simulink model "train_fuzzy4"  (R2017b)
settings: Solver=FixedStepAuto  StartTime=0.0  StopTime=1000  FixedStep=0.01  RelTol=1e-3
libraries: fuzblock x1
settings Model: Creator=QuocViet  LastModifiedBy=QuocViet
settings DebuggingCC: UnconnectedInputMsg=none  UnconnectedOutputMsg=none  UnconnectedLineMsg=none  SFMachineParentedDataDiag=error
settings SFSimCC: SimUseLocalCustomCode=on
settings RTWCC: RTWUseLocalCustomCode=on

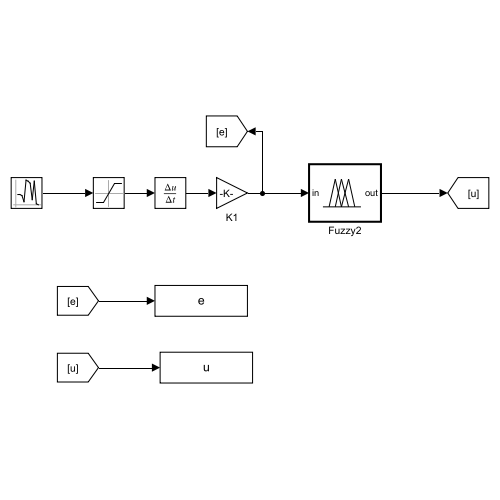
[thumbnail: Simulink's stored preview of the top-level diagram]
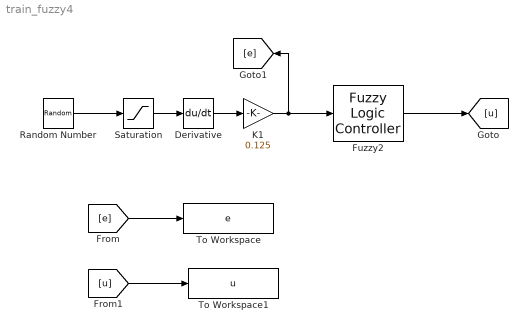
== system train_fuzzy4 ==
  Derivative : Derivative
  Fuzzy2 : fuzblock/Fuzzy Logic  Controller  FIS='RULE222.fis'  OutputSampleNumber=101  DataType=double  FuzzifiedInputs=off  RuleFiringStrengths=off  RuleOutputs=off  AggregatedOutputs=off  SimulateUsing=Interpreted execution  OutOfRangeInputValueMessage=warning  NoRuleFiredMessage=warning  EmptyOutputFuzzySetMessage=warning
  K1 : Gain  Gain=0.125
  Random Number : RandomNumber  Variance=0.01  SampleTime=0.1
  Saturation : Saturate  UpperLimit=0.01  LowerLimit=-0.01
  To Workspace : ToWorkspace  VariableName=e  SampleTime=-1
  To Workspace1 : ToWorkspace  VariableName=u  SampleTime=-1
  wires:
  Random Number/1 -> Saturation/1
  K1/1 -> Fuzzy2/1, [e]
  Fuzzy2/1 -> [u]
  [e] -> To Workspace/1
  [u] -> To Workspace1/1
  Saturation/1 -> Derivative/1
  Derivative/1 -> K1/1
